simulink model "stabilitate2"  (R2024a)
settings: Solver=VariableStepAuto  StartTime=0.0  StopTime=1000  RelTol=1e-3
values from neighbouring files (symbols this model uses):
  k = -0.9    [parametrii.m]
settings Model: Creator=paulhondola  LastModifiedBy=paulhondola

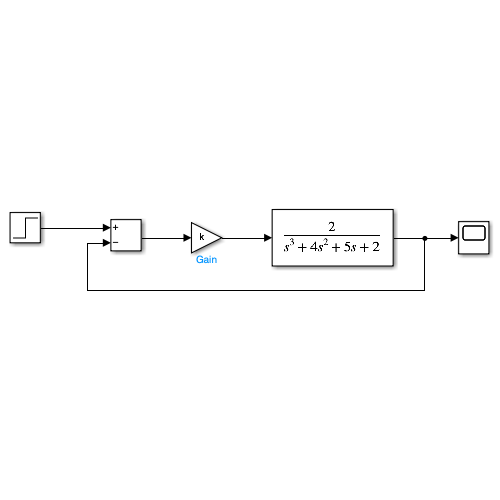
[thumbnail: Simulink's stored preview of the top-level diagram]
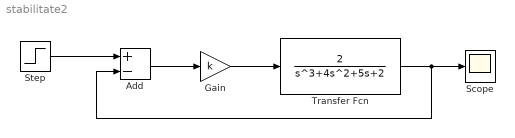
== system stabilitate2 ==
  Add : Sum  Inputs=+-
  Gain : Gain  Gain=k
  Scope : Scope
  Step : Step  After=10  SampleTime=0
  Transfer Fcn : TransferFcn  Numerator=[2]  Denominator=[1 4 5 2]
  wires:
  Gain/1 -> Transfer Fcn/1
  Transfer Fcn/1 -> Add/2, Scope/1
  Step/1 -> Add/1
  Add/1 -> Gain/1
